simulink model "fake_config"  (R2017b)
settings: Solver=VariableStepAuto  StartTime=0.0  StopTime=10.0  RelTol=1e-3
libraries: simulink_extras x18
(part 1 of 4)
settings Model: Creator=Tonno  LastModifiedBy=Tonno

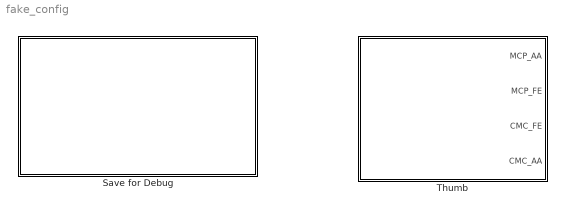
== system fake_config ==
  Save for Debug : Subsystem
  Thumb : Subsystem

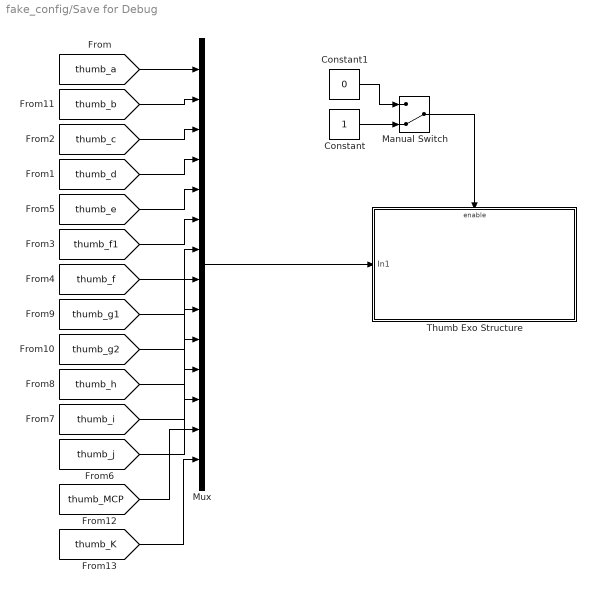
== system fake_config/Save for Debug ==
  Constant : Constant
  Constant1 : Constant  Value=0
  Manual Switch : ManualSwitch  CurrentSetting=0
  Mux : Mux  Inputs=14
  Thumb Exo Structure : Subsystem
  wires:
  Manual Switch/1 -> Thumb Exo Structure/Enable
  Constant/1 -> Manual Switch/2
  Constant1/1 -> Manual Switch/1
  [thumb_i] -> Mux/11
  [thumb_g2] -> Mux/9
  [thumb_c] -> Mux/3
  [thumb_d] -> Mux/4
  [thumb_f] -> Mux/7
  [thumb_f1] -> Mux/6
  [thumb_h] -> Mux/10
  [thumb_b] -> Mux/2
  Mux/1 -> Thumb Exo Structure/1(In1)
  [thumb_j] -> Mux/12
  [thumb_a] -> Mux/1
  [thumb_e] -> Mux/5
  [thumb_g1] -> Mux/8
  [thumb_MCP] -> Mux/13
  [thumb_K] -> Mux/14

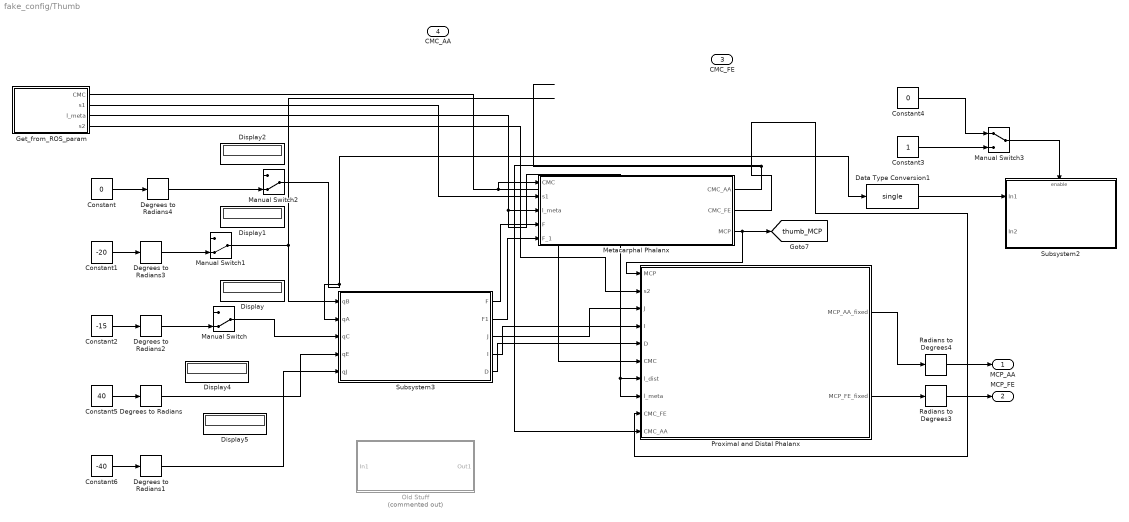
== system fake_config/Thumb ==
  Constant : Constant  Value=0
  Constant1 : Constant  Value=-20
  Constant2 : Constant  Value=-15
  Constant3 : Constant
  Constant4 : Constant  Value=0
  Constant5 : Constant  Value=40
  Constant6 : Constant  Value=-40
  Data Type Conversion1 : DataTypeConversion  OutDataTypeStr=single
  Degrees to Radians{,1..4} (5 alike) : simulink_extras/Transformations/Degrees to Radians
  Display{,1..2,4..5} (5 alike) : Display
  Get_from_ROS_param : Subsystem
  Manual Switch : ManualSwitch  CurrentSetting=0
  Manual Switch1 : ManualSwitch  CurrentSetting=0
  Manual Switch2 : ManualSwitch  CurrentSetting=0
  Manual Switch3 : ManualSwitch
  Metacarphal Phalanx : Subsystem
  Old Stuff : Subsystem  Commented=on
  Proximal and Distal Phalanx : Subsystem
  Radians to Degrees3 : simulink_extras/Transformations/Radians to Degrees
  Radians to Degrees4 : simulink_extras/Transformations/Radians to Degrees
  Subsystem2 : Subsystem
  Subsystem3 : Subsystem
  MCP_AA : Outport
  MCP_FE : Outport  Port=2
  CMC_FE : Outport  Port=3
  CMC_AA : Outport  Port=4
  tag scope: thumb_MCP=global
  wires:
  Constant2/1 -> Degrees to Radians2/1
  Constant1/1 -> Degrees to Radians3/1
  Constant/1 -> Degrees to Radians4/1
  Get_from_ROS_param/1(CMC) -> Proximal and Distal Phalanx/6(CMC), Metacarphal Phalanx/1(CMC)
  Get_from_ROS_param/2(s1) -> Metacarphal Phalanx/2(s1)
  Metacarphal Phalanx/3(MCP) -> [thumb_MCP], Proximal and Distal Phalanx/1("MCP ")
  Get_from_ROS_param/3(l_meta) -> Proximal and Distal Phalanx/7(l_dist), Proximal and Distal Phalanx/8(l_meta), Metacarphal Phalanx/3(l_meta)
  Get_from_ROS_param/4(s2) -> Proximal and Distal Phalanx/2(s2)
  Proximal and Distal Phalanx/1(MCP_AA_fixed) -> Radians to Degrees4/1
  Radians to Degrees3/1 -> MCP_FE/1
  Proximal and Distal Phalanx/2(MCP_FE_fixed) -> Radians to Degrees3/1
  Radians to Degrees4/1 -> MCP_AA/1
  Manual Switch2/1 -> Data Type Conversion1/1, Subsystem3/2(qA)
  Manual Switch1/1 -> Subsystem3/1(qB)
  Metacarphal Phalanx/2(CMC_FE) -> Proximal and Distal Phalanx/9(CMC_FE)
  Metacarphal Phalanx/1("CMC_AA ") -> Proximal and Distal Phalanx/10(CMC_AA)
  Manual Switch3/1 -> Subsystem2/Enable
  Constant3/1 -> Manual Switch3/2
  Constant4/1 -> Manual Switch3/1
  Data Type Conversion1/1 -> Subsystem2/1(In1)
  Manual Switch/1 -> Subsystem3/3(qC)
  Subsystem3/1(F) -> Metacarphal Phalanx/4(F)
  Subsystem3/2(F1) -> Metacarphal Phalanx/5(F_1)
  Subsystem3/3(J) -> Proximal and Distal Phalanx/3(J)
  Subsystem3/4(I) -> Proximal and Distal Phalanx/4(I)
  Subsystem3/5(D) -> Proximal and Distal Phalanx/5(D)
  ? -> CMC_FE/1
  ? -> CMC_AA/1
  Constant5/1 -> Degrees to Radians/1
  Constant6/1 -> Degrees to Radians1/1
  Degrees to Radians1/1 -> Subsystem3/5(qJ)
  Degrees to Radians/1 -> Subsystem3/4(qE)
  Degrees to Radians2/1 -> Manual Switch/2
  Degrees to Radians3/1 -> Manual Switch1/2
  Degrees to Radians4/1 -> Manual Switch2/2

== system fake_config/Save for Debug/Thumb Exo Structure ==
  In1 : Inport
  Enable : EnablePort
  Data Type Conversion1 : DataTypeConversion  OutDataTypeStr=double
  To File : ToFile  Filename=exo_points.mat  MatrixName=points
  wires:
  In1/1 -> Data Type Conversion1/1
  Data Type Conversion1/1 -> To File/1

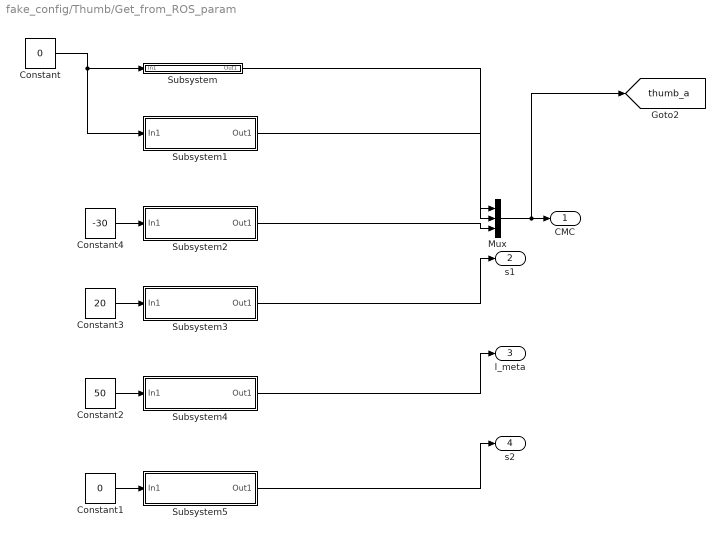
== system fake_config/Thumb/Get_from_ROS_param ==
  Constant : Constant  Value=0
  Constant1 : Constant  Value=0
  Constant2 : Constant  Value=50
  Constant3 : Constant  Value=20
  Constant4 : Constant  Value=-30
  Mux : Mux  Inputs=3
  Subsystem : Subsystem
  Subsystem1 : Subsystem
  Subsystem2 : Subsystem
  Subsystem3 : Subsystem
  Subsystem4 : Subsystem
  Subsystem5 : Subsystem
  CMC : Outport
  s1 : Outport  Port=2
  l_meta : Outport  Port=3
  s2 : Outport  Port=4
  tag scope: thumb_a=global
  wires:
  Mux/1 -> [thumb_a], CMC/1
  Subsystem/1(Out1) -> Mux/1
  Subsystem1/1(Out1) -> Mux/2
  Subsystem2/1(Out1) -> Mux/3
  Subsystem3/1(Out1) -> s1/1
  Subsystem4/1(Out1) -> l_meta/1
  Subsystem5/1(Out1) -> s2/1
  Constant/1 -> Subsystem1/1(In1), Subsystem/1(In1)
  Constant3/1 -> Subsystem3/1(In1)
  Constant2/1 -> Subsystem4/1(In1)
  Constant1/1 -> Subsystem5/1(In1)
  Constant4/1 -> Subsystem2/1(In1)

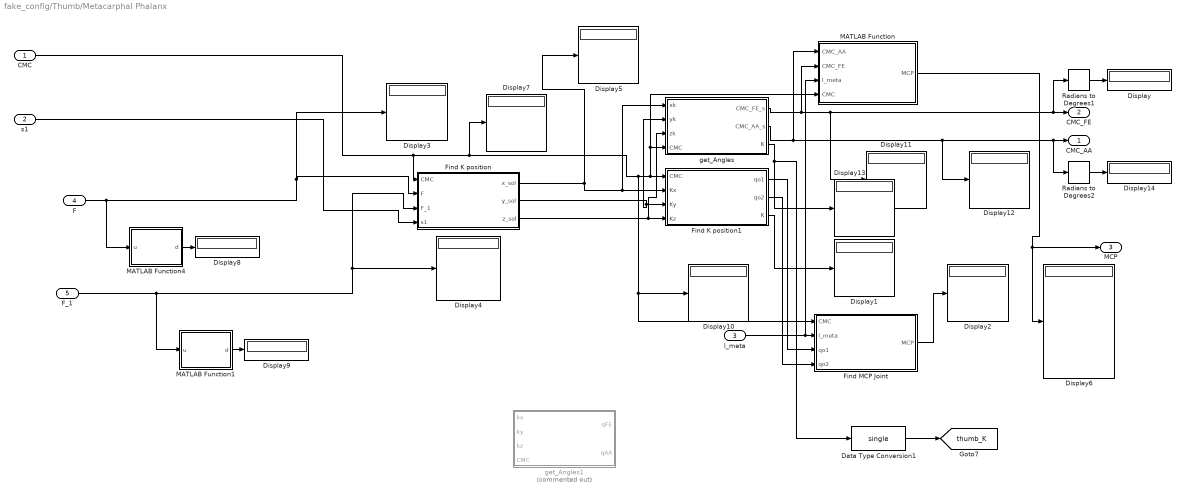
== system fake_config/Thumb/Metacarphal Phalanx ==
  CMC : Inport
  s1 : Inport  Port=2
  l_meta : Inport  Port=3
  F : Inport  Port=4
  F_1 : Inport  Port=5
  Data Type Conversion1 : DataTypeConversion  OutDataTypeStr=single
  Display{,1..14} (15 alike) : Display
  Find K position : MATLAB Function  TreatAsAtomicUnit=on
  Find K position1 : MATLAB Function  TreatAsAtomicUnit=on
  Find MCP Joint : MATLAB Function  TreatAsAtomicUnit=on
  MATLAB Function : MATLAB Function  TreatAsAtomicUnit=on
  MATLAB Function1 : MATLAB Function  TreatAsAtomicUnit=on
  MATLAB Function4 : MATLAB Function  TreatAsAtomicUnit=on
  Radians to Degrees1 : simulink_extras/Transformations/Radians to Degrees
  Radians to Degrees2 : simulink_extras/Transformations/Radians to Degrees
  get_Angles : MATLAB Function  TreatAsAtomicUnit=on
  get_Angles1 : MATLAB Function  Commented=on  TreatAsAtomicUnit=on
  "CMC_AA " : Outport
  CMC_FE : Outport  Port=2
  MCP : Outport  Port=3
  tag scope: thumb_K=global
  wires:
  Find K position/2(y_sol) -> get_Angles/2(yk), Find K position1/3(Ky)
  Find K position1/1(qo1) -> Find MCP Joint/3(qo1)
  Find K position1/2(qo2) -> Find MCP Joint/4(qo2)
  Find K position/3(z_sol) -> get_Angles/3(zk), Find K position1/4(Kz)
  Find K position/1(x_sol) -> Display5/1, get_Angles/1(xk), Find K position1/2(Kx)
  CMC/1 -> Display7/1, Display10/1, Find MCP Joint/1(CMC), MATLAB Function/4(CMC), get_Angles/4(CMC), Find K position1/1(CMC), Find K position/1(CMC)
  s1/1 -> Find K position/4(s1)
  l_meta/1 -> MATLAB Function/3(l_meta), Find MCP Joint/2(l_meta)
  Find MCP Joint/1(MCP) -> Display2/1
  Find K position1/3(K) -> Display1/1
  get_Angles/2(CMC_AA_s) -> MATLAB Function/1(CMC_AA), Display12/1, Radians to Degrees2/1, "CMC_AA "/1
  get_Angles/1(CMC_FE_s) -> MATLAB Function/2(CMC_FE), Display11/1, Radians to Degrees1/1, CMC_FE/1
  MATLAB Function4/1(d) -> Display8/1
  F/1 -> MATLAB Function4/1(u), Find K position/2(F), Display3/1
  MATLAB Function1/1(d) -> Display9/1
  F_1/1 -> MATLAB Function1/1(u), Find K position/3(F_1), Display4/1
  MATLAB Function/1(MCP) -> MCP/1, Display6/1
  get_Angles/3(K) -> Data Type Conversion1/1, Display13/1
  Radians to Degrees1/1 -> Display/1
  Radians to Degrees2/1 -> Display14/1
  Data Type Conversion1/1 -> [thumb_K]

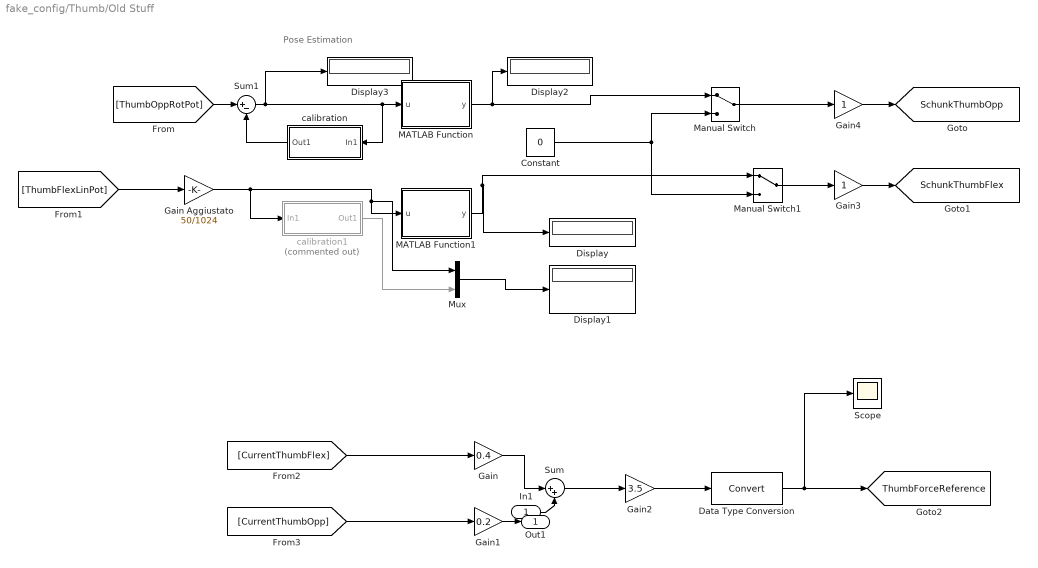
== system fake_config/Thumb/Old Stuff ==
  note: Pose Estimation
  In1 : Inport
  Constant : Constant  Value=0  OutDataTypeStr=single
  Data Type Conversion : DataTypeConversion
  Display{,1..3} (4 alike) : Display
  Gain : Gain  Gain=0.4
  Gain Aggiustato : Gain  Gain=50/1024
  Gain1 : Gain  Gain=0.2
  Gain2 : Gain  Gain=3.5
  Gain3 : Gain
  Gain4 : Gain
  MATLAB Function : MATLAB Function  TreatAsAtomicUnit=on
  MATLAB Function1 : MATLAB Function  TreatAsAtomicUnit=on
  Manual Switch : ManualSwitch
  Manual Switch1 : ManualSwitch
  Mux : Mux  Inputs=2
  Scope : Scope
  Sum : Sum  Inputs=|++
  Sum1 : Sum  Inputs=|+-
  calibration : Subsystem
  calibration1 : Subsystem  Commented=on
  Out1 : Outport
  tag scope: SchunkThumbFlex=global, SchunkThumbOpp=global, ThumbForceReference=global
  wires:
  Gain1/1 -> Out1/1
  In1/1 -> Sum/2
  MATLAB Function/1(y) -> Display2/1, Manual Switch/1
  Gain4/1 -> [SchunkThumbOpp]
  [ThumbFlexLinPot] -> Gain Aggiustato/1
  Sum/1 -> Gain2/1
  Data Type Conversion/1 -> Scope/1, [ThumbForceReference]
  Gain2/1 -> Data Type Conversion/1
  Gain3/1 -> [SchunkThumbFlex]
  Sum1/1 -> Display3/1, calibration/1(In1), MATLAB Function/1(u)
  Mux/1 -> Display1/1
  [CurrentThumbFlex] -> Gain/1
  MATLAB Function1/1(y) -> Manual Switch1/1, Display/1
  Manual Switch/1 -> Gain4/1
  Manual Switch1/1 -> Gain3/1
  [CurrentThumbOpp] -> Gain1/1
  Constant/1 -> Manual Switch1/2, Manual Switch/2
  calibration/1(Out1) -> Sum1/2
  Gain/1 -> Sum/1
  calibration1/1(Out1) -> Mux/2
  Gain Aggiustato/1 -> calibration1/1(In1), Mux/1, MATLAB Function1/1(u)
  [ThumbOppRotPot] -> Sum1/1

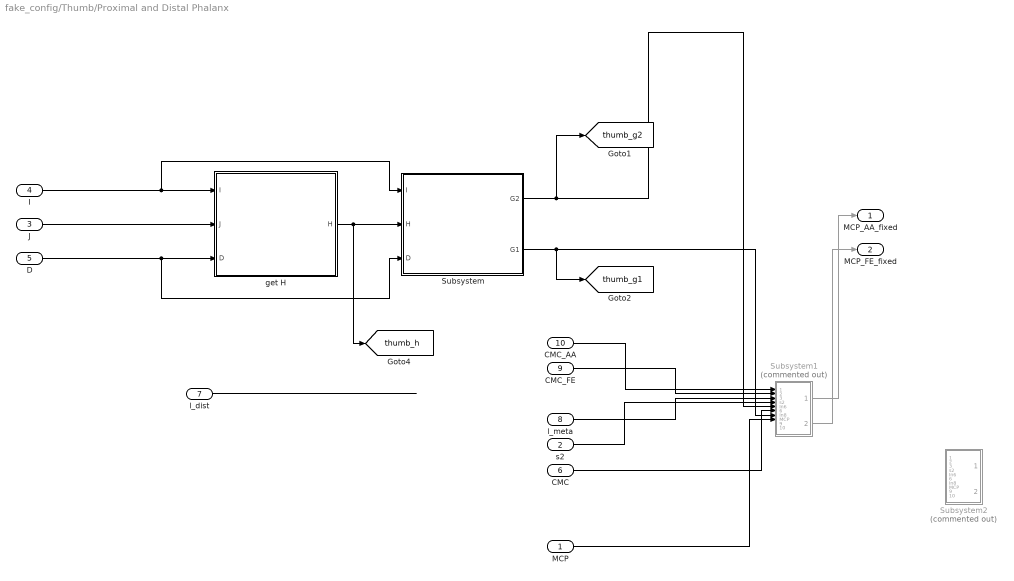
== system fake_config/Thumb/Proximal and Distal Phalanx ==
  "MCP " : Inport
  s2 : Inport  Port=2
  J : Inport  Port=3
  I : Inport  Port=4
  D : Inport  Port=5
  CMC : Inport  Port=6
  l_dist : Inport  Port=7
  l_meta : Inport  Port=8
  CMC_FE : Inport  Port=9
  CMC_AA : Inport  Port=10
  Subsystem : Subsystem
  Subsystem1 : Subsystem  Commented=on
  Subsystem2 : Subsystem  Commented=on
  get H : Subsystem
  MCP_AA_fixed : Outport
  MCP_FE_fixed : Outport  Port=2
  tag scope: thumb_g1=global, thumb_g2=global, thumb_h=global
  wires:
  I/1 -> Subsystem/1(I), get H/1(I)
  J/1 -> get H/2(J)
  D/1 -> Subsystem/3(D), get H/3(D)
  get H/1(H) -> [thumb_h], Subsystem/2(H)
  CMC_AA/1 -> Subsystem1/1(CMC_AA)
  CMC_FE/1 -> Subsystem1/2(CMC_FE)
  l_dist/1 -> ?
  l_meta/1 -> Subsystem1/3(l_meta)
  s2/1 -> Subsystem1/4(s2)
  Subsystem/1(G2) -> [thumb_g2], Subsystem1/5(In6)
  CMC/1 -> Subsystem1/6(CMC)
  Subsystem/2(G1) -> [thumb_g1], Subsystem1/7(In8)
  "MCP "/1 -> Subsystem1/8("MCP ")
  Subsystem1/1(MCP_AA_fixed) -> MCP_AA_fixed/1
  Subsystem1/2(MCP_FE_fixed) -> MCP_FE_fixed/1

== system fake_config/Thumb/Subsystem2 ==
  In1 : Inport
  In2 : Inport  Port=2
  Enable : EnablePort
  Data Type Conversion1 : DataTypeConversion  OutDataTypeStr=double
  Mux : Mux  Inputs=2
  To File : ToFile  Filename=thumb_force.mat  MatrixName=forza_gravita
  wires:
  In1/1 -> Mux/1
  Mux/1 -> Data Type Conversion1/1
  In2/1 -> Mux/2
  Data Type Conversion1/1 -> To File/1

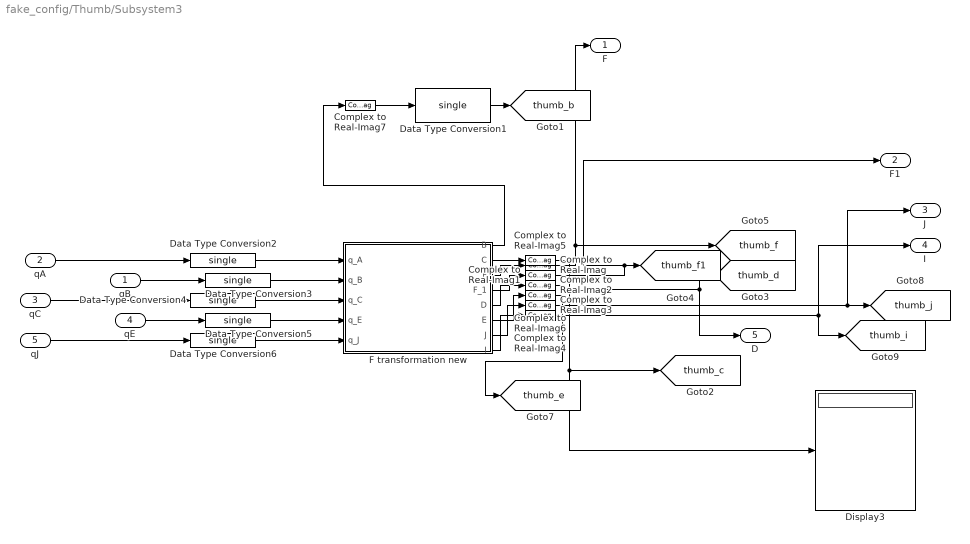
== system fake_config/Thumb/Subsystem3 ==
  qB : Inport
  qA : Inport  Port=2
  qC : Inport  Port=3
  qE : Inport  Port=4
  qJ : Inport  Port=5
  Complex to Real-Imag{,1..7} (8 alike) : ComplexToRealImag  Output=Real
  Data Type Conversion{1..6} (6 alike) : DataTypeConversion  OutDataTypeStr=single
  Display3 : Display
  F transformation new : MATLAB Function  TreatAsAtomicUnit=on
  F : Outport
  F1 : Outport  Port=2
  J : Outport  Port=3
  I : Outport  Port=4
  D : Outport  Port=5
  tag scope: thumb_b=global, thumb_c=global, thumb_d=global, thumb_e=global, thumb_f1=global, thumb_f=global, thumb_i=global, thumb_j=global
  wires:
  Complex to Real-Imag5/1 -> Display3/1, [thumb_c]
  qA/1 -> Data Type Conversion2/1
  Complex to Real-Imag6/1 -> [thumb_e]
  F transformation new/6(E) -> Complex to Real-Imag6/1
  F transformation new/1(B) -> Complex to Real-Imag7/1
  qE/1 -> Data Type Conversion5/1
  qB/1 -> Data Type Conversion3/1
  qC/1 -> Data Type Conversion4/1
  F transformation new/3(F) -> Complex to Real-Imag/1
  F transformation new/4(F_1) -> Complex to Real-Imag1/1
  F transformation new/7(J) -> Complex to Real-Imag3/1
  F transformation new/8(I) -> Complex to Real-Imag4/1
  F transformation new/5(D) -> Complex to Real-Imag2/1
  Complex to Real-Imag/1 -> F/1, [thumb_f]
  Complex to Real-Imag1/1 -> F1/1, [thumb_f1]
  Complex to Real-Imag2/1 -> D/1, [thumb_d]
  Complex to Real-Imag3/1 -> J/1, [thumb_j]
  Complex to Real-Imag4/1 -> I/1, [thumb_i]
  F transformation new/2(C) -> Complex to Real-Imag5/1
  Complex to Real-Imag7/1 -> Data Type Conversion1/1
  Data Type Conversion1/1 -> [thumb_b]
  Data Type Conversion2/1 -> F transformation new/1(q_A)
  Data Type Conversion3/1 -> F transformation new/2(q_B)
  Data Type Conversion4/1 -> F transformation new/3(q_C)
  Data Type Conversion5/1 -> F transformation new/4(q_E)
  Data Type Conversion6/1 -> F transformation new/5(q_J)
  qJ/1 -> Data Type Conversion6/1

== system fake_config/Thumb/Get_from_ROS_param/Subsystem ==
  In1 : Inport
  Data Type Conversion1 : DataTypeConversion  OutDataTypeStr=single
  Rate Transition : RateTransition  InitialCondition=-10.0
  Out1 : Outport
  wires:
  Data Type Conversion1/1 -> Out1/1
  In1/1 -> Rate Transition/1
  Rate Transition/1 -> Data Type Conversion1/1

== system fake_config/Thumb/Get_from_ROS_param/Subsystem1 ==
  In1 : Inport
  Data Type Conversion1 : DataTypeConversion  OutDataTypeStr=single
  Rate Transition : RateTransition  InitialCondition=0.0
  Out1 : Outport
  wires:
  Data Type Conversion1/1 -> Out1/1
  In1/1 -> Rate Transition/1
  Rate Transition/1 -> Data Type Conversion1/1

== system fake_config/Thumb/Get_from_ROS_param/Subsystem2 ==
  In1 : Inport
  Data Type Conversion1 : DataTypeConversion  OutDataTypeStr=single
  Rate Transition : RateTransition  InitialCondition=-32.0
  Out1 : Outport
  wires:
  Data Type Conversion1/1 -> Out1/1
  In1/1 -> Rate Transition/1
  Rate Transition/1 -> Data Type Conversion1/1

== system fake_config/Thumb/Get_from_ROS_param/Subsystem3 ==
  In1 : Inport
  Data Type Conversion1 : DataTypeConversion  OutDataTypeStr=single
  Rate Transition : RateTransition  InitialCondition=20.0
  Out1 : Outport
  wires:
  Data Type Conversion1/1 -> Out1/1
  In1/1 -> Rate Transition/1
  Rate Transition/1 -> Data Type Conversion1/1

== system fake_config/Thumb/Get_from_ROS_param/Subsystem4 ==
  In1 : Inport
  Data Type Conversion1 : DataTypeConversion  OutDataTypeStr=single
  Rate Transition : RateTransition  InitialCondition=50.0
  Out1 : Outport
  wires:
  Data Type Conversion1/1 -> Out1/1
  In1/1 -> Rate Transition/1
  Rate Transition/1 -> Data Type Conversion1/1

== system fake_config/Thumb/Get_from_ROS_param/Subsystem5 ==
  In1 : Inport
  Data Type Conversion1 : DataTypeConversion  OutDataTypeStr=single
  Rate Transition : RateTransition  InitialCondition=20.0
  Out1 : Outport
  wires:
  Data Type Conversion1/1 -> Out1/1
  In1/1 -> Rate Transition/1
  Rate Transition/1 -> Data Type Conversion1/1

== system fake_config/Thumb/Old Stuff/calibration ==
  In1 : Inport
  Constant2 : Constant  Value=540  OutDataTypeStr=single
  Constant3 : Constant  Value=540  OutDataTypeStr=single
  Display4 : Display
  Subsystem : Subsystem
  Sum2 : Sum  Inputs=|++
  Switch : Switch  Criteria=u2 > Threshold
  Out1 : Outport
  wires:
  [CalibrationSignal] -> Switch/2
  Subsystem/1(Out1) -> Switch/3
  Constant3/1 -> Sum2/1
  [CalibrationSignal] -> Subsystem/Enable
  Constant2/1 -> Switch/1
  Sum2/1 -> Display4/1, Subsystem/1(In1)
  In1/1 -> Sum2/2
  Switch/1 -> Out1/1

== system fake_config/Thumb/Old Stuff/calibration1 ==
  In1 : Inport
  Subsystem1 : Subsystem
  Out1 : Outport
  wires:
  [CalibrationSignal] -> Subsystem1/Enable
  In1/1 -> Subsystem1/1(In1)
  Subsystem1/1(Out1) -> Out1/1

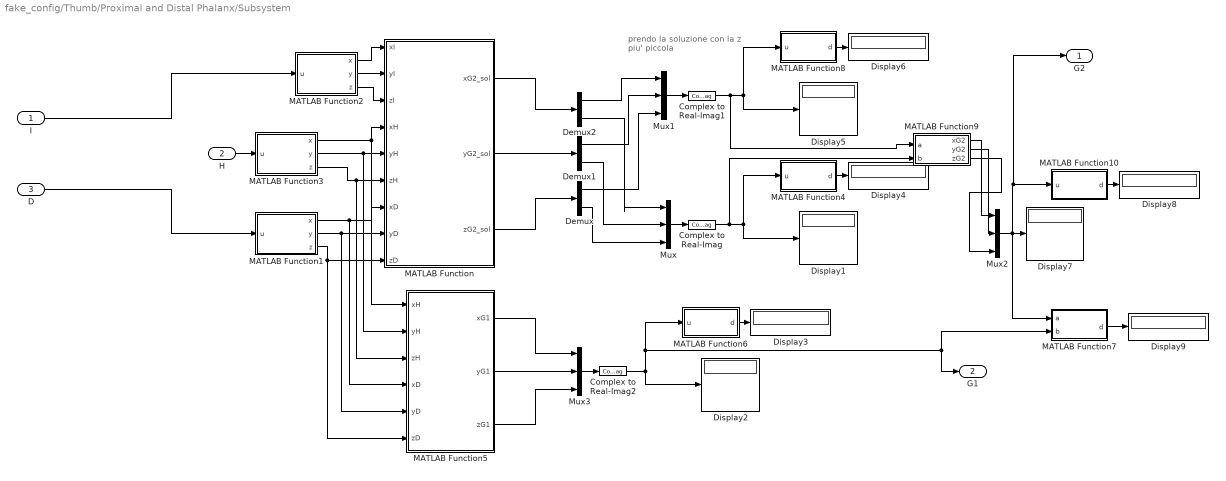
== system fake_config/Thumb/Proximal and Distal Phalanx/Subsystem ==
  note: prendo la soluzione
      | con la z piu' piccola
  I : Inport
  H : Inport  Port=2
  D : Inport  Port=3
  Complex to Real-Imag : ComplexToRealImag  Output=Real
  Complex to Real-Imag1 : ComplexToRealImag  Output=Real
  Complex to Real-Imag2 : ComplexToRealImag  Output=Real
  Demux : Demux  Outputs=2
  Demux1 : Demux  Outputs=2
  Demux2 : Demux  Outputs=2
  Display{1..9} (9 alike) : Display
  MATLAB Function : MATLAB Function  TreatAsAtomicUnit=on
  MATLAB Function1 : MATLAB Function  TreatAsAtomicUnit=on
  MATLAB Function10 : MATLAB Function  TreatAsAtomicUnit=on
  MATLAB Function2 : MATLAB Function  TreatAsAtomicUnit=on
  MATLAB Function3 : MATLAB Function  TreatAsAtomicUnit=on
  MATLAB Function4 : MATLAB Function  TreatAsAtomicUnit=on
  MATLAB Function5 : MATLAB Function  TreatAsAtomicUnit=on
  MATLAB Function6 : MATLAB Function  TreatAsAtomicUnit=on
  MATLAB Function7 : MATLAB Function  TreatAsAtomicUnit=on
  MATLAB Function8 : MATLAB Function  TreatAsAtomicUnit=on
  MATLAB Function9 : MATLAB Function  TreatAsAtomicUnit=on
  Mux{,1..3} (4 alike) : Mux  Inputs=3
  G2 : Outport
  G1 : Outport  Port=2
  wires:
  MATLAB Function1/2(y) -> MATLAB Function/8(yD), MATLAB Function5/5(yD)
  H/1 -> MATLAB Function3/1(u)
  MATLAB Function3/1(x) -> MATLAB Function5/1(xH), MATLAB Function/4(xH)
  MATLAB Function2/1(x) -> MATLAB Function/1(xI)
  D/1 -> MATLAB Function1/1(u)
  MATLAB Function/1(xG2_sol) -> Demux2/1
  Complex to Real-Imag1/1 -> MATLAB Function9/1(a), Display5/1, MATLAB Function8/1(u)
  Demux/2 -> Mux/3
  MATLAB Function10/1(d) -> Display8/1
  MATLAB Function/3(zG2_sol) -> Demux/1
  MATLAB Function2/3(z) -> MATLAB Function/3(zI)
  MATLAB Function2/2(y) -> MATLAB Function/2(yI)
  MATLAB Function9/3(zG2) -> Mux2/3
  Demux2/1 -> Mux1/1
  MATLAB Function1/3(z) -> MATLAB Function5/6(zD), MATLAB Function/9(zD)
  MATLAB Function9/1(xG2) -> Mux2/1
  Demux1/1 -> Mux1/2
  MATLAB Function1/1(x) -> MATLAB Function/7(xD), MATLAB Function5/4(xD)
  Complex to Real-Imag/1 -> MATLAB Function9/2(b), Display1/1, MATLAB Function4/1(u)
  Demux2/2 -> Mux/1
  MATLAB Function9/2(yG2) -> Mux2/2
  I/1 -> MATLAB Function2/1(u)
  Demux/1 -> Mux1/3
  Mux1/1 -> Complex to Real-Imag1/1
  Mux/1 -> Complex to Real-Imag/1
  MATLAB Function3/2(y) -> MATLAB Function5/2(yH), MATLAB Function/5(yH)
  MATLAB Function4/1(d) -> Display4/1
  MATLAB Function3/3(z) -> MATLAB Function/6(zH), MATLAB Function5/3(zH)
  Demux1/2 -> Mux/2
  MATLAB Function/2(yG2_sol) -> Demux1/1
  MATLAB Function8/1(d) -> Display6/1
  Mux3/1 -> Complex to Real-Imag2/1
  MATLAB Function5/2(yG1) -> Mux3/2
  MATLAB Function5/1(xG1) -> Mux3/1
  MATLAB Function5/3(zG1) -> Mux3/3
  MATLAB Function6/1(d) -> Display3/1
  Complex to Real-Imag2/1 -> Display2/1, G1/1, MATLAB Function7/2(b), MATLAB Function6/1(u)
  Mux2/1 -> MATLAB Function7/1(a), G2/1, MATLAB Function10/1(u), Display7/1
  MATLAB Function7/1(d) -> Display9/1

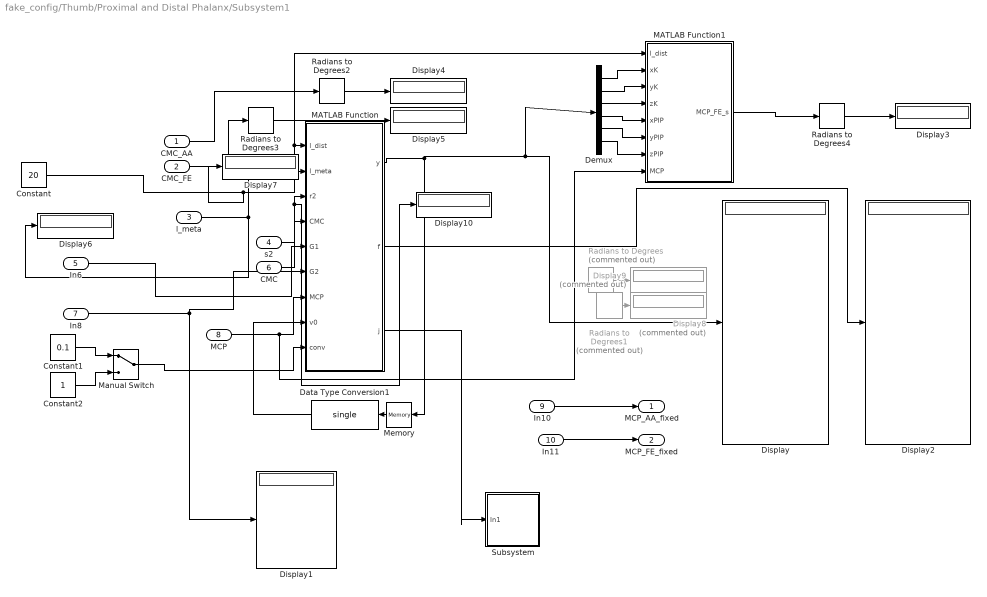
== system fake_config/Thumb/Proximal and Distal Phalanx/Subsystem1 ==
  CMC_AA : Inport
  CMC_FE : Inport  Port=2
  l_meta : Inport  Port=3
  s2 : Inport  Port=4
  In6 : Inport  Port=5
  CMC : Inport  Port=6
  In8 : Inport  Port=7
  "MCP " : Inport  Port=8
  In10 : Inport  Port=9
  In11 : Inport  Port=10
  Constant : Constant  Value=20  OutDataTypeStr=single
  Constant1 : Constant  Value=0.1  OutDataTypeStr=single
  Constant2 : Constant  OutDataTypeStr=single
  Data Type Conversion1 : DataTypeConversion  OutDataTypeStr=single
  Demux : Demux  Outputs=6
  Display{,1..7,10} (9 alike) : Display
  Display8 : Display  Commented=on
  Display9 : Display  Commented=on
  MATLAB Function : MATLAB Function  TreatAsAtomicUnit=on
  MATLAB Function1 : MATLAB Function  TreatAsAtomicUnit=on
  Manual Switch : ManualSwitch
  Memory : Memory
  Radians to Degrees : simulink_extras/Transformations/Radians to Degrees  Commented=on
  Radians to Degrees1 : simulink_extras/Transformations/Radians to Degrees  Commented=on
  Radians to Degrees2 : simulink_extras/Transformations/Radians to Degrees
  Radians to Degrees3 : simulink_extras/Transformations/Radians to Degrees
  Radians to Degrees4 : simulink_extras/Transformations/Radians to Degrees
  Subsystem : Subsystem
  MCP_AA_fixed : Outport
  MCP_FE_fixed : Outport  Port=2
  wires:
  ? -> Radians to Degrees1/1
  MATLAB Function/2(f) -> Display2/1
  Memory/1 -> Data Type Conversion1/1
  Data Type Conversion1/1 -> MATLAB Function/8(v0)
  Radians to Degrees1/1 -> Display8/1
  CMC_AA/1 -> Radians to Degrees2/1
  MATLAB Function/1(y) -> Demux/1, Display/1, Memory/1
  Radians to Degrees/1 -> Display9/1
  s2/1 -> Display10/1, MATLAB Function/3(r2)
  In8/1 -> MATLAB Function/6(G2), Display1/1
  CMC_FE/1 -> Radians to Degrees3/1
  "MCP "/1 -> MATLAB Function1/8(MCP), MATLAB Function/7(MCP)
  ? -> Radians to Degrees/1
  In10/1 -> MCP_AA_fixed/1
  In11/1 -> MCP_FE_fixed/1
  In6/1 -> MATLAB Function/5(G1)
  CMC/1 -> MATLAB Function/4(CMC)
  l_meta/1 -> Display6/1, MATLAB Function/2(l_meta)
  Constant/1 -> Display7/1, MATLAB Function1/1(l_dist), MATLAB Function/1(l_dist)
  MATLAB Function/3(j) -> Subsystem/1(In1)
  Radians to Degrees2/1 -> Display4/1
  Radians to Degrees3/1 -> Display5/1
  MATLAB Function1/1(MCP_FE_s) -> Radians to Degrees4/1
  Demux/6 -> MATLAB Function1/7(zPIP)
  Demux/5 -> MATLAB Function1/6(yPIP)
  Demux/4 -> MATLAB Function1/5(xPIP)
  Demux/3 -> MATLAB Function1/4(zK)
  Demux/2 -> MATLAB Function1/3(yK)
  Demux/1 -> MATLAB Function1/2(xK)
  Radians to Degrees4/1 -> Display3/1
  Manual Switch/1 -> MATLAB Function/9(conv)
  Constant1/1 -> Manual Switch/1
  Constant2/1 -> Manual Switch/2

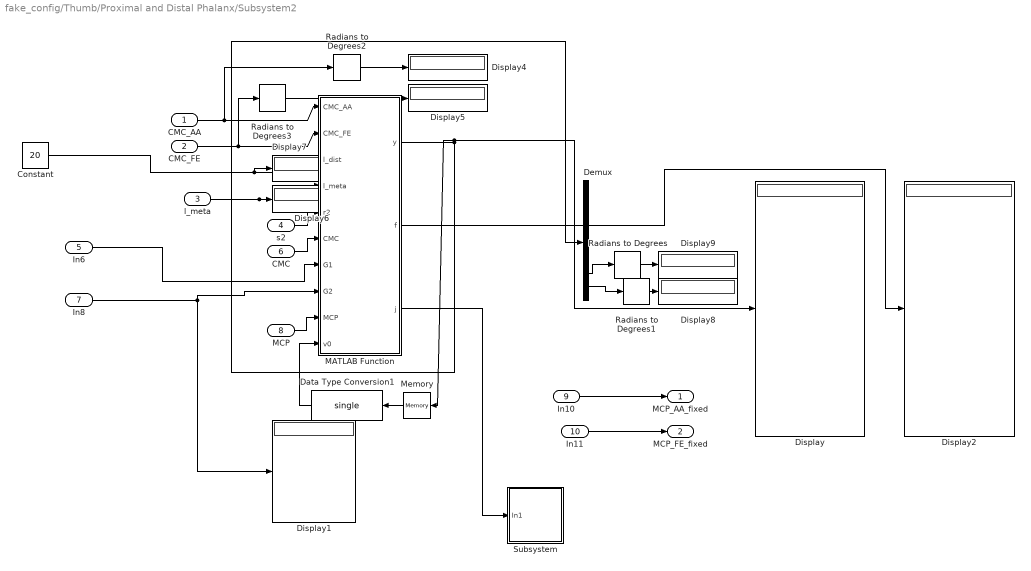
== system fake_config/Thumb/Proximal and Distal Phalanx/Subsystem2 ==
  CMC_AA : Inport
  CMC_FE : Inport  Port=2
  l_meta : Inport  Port=3
  s2 : Inport  Port=4
  In6 : Inport  Port=5
  CMC : Inport  Port=6
  In8 : Inport  Port=7
  "MCP " : Inport  Port=8
  In10 : Inport  Port=9
  In11 : Inport  Port=10
  Constant : Constant  Value=20  OutDataTypeStr=single
  Data Type Conversion1 : DataTypeConversion  OutDataTypeStr=single
  Demux : Demux  Outputs=8
  Display{,1..2,4..9} (9 alike) : Display
  MATLAB Function : MATLAB Function  TreatAsAtomicUnit=on
  Memory : Memory
  Radians to Degrees{,1..3} (4 alike) : simulink_extras/Transformations/Radians to Degrees
  Subsystem : Subsystem
  MCP_AA_fixed : Outport
  MCP_FE_fixed : Outport  Port=2
  wires:
  Demux/8 -> Radians to Degrees1/1
  MATLAB Function/2(f) -> Display2/1
  Memory/1 -> Data Type Conversion1/1
  Data Type Conversion1/1 -> MATLAB Function/10(v0)
  Radians to Degrees1/1 -> Display8/1
  CMC_AA/1 -> Radians to Degrees2/1, MATLAB Function/1(CMC_AA)
  MATLAB Function/1(y) -> Memory/1, Display/1, Demux/1
  Radians to Degrees/1 -> Display9/1
  s2/1 -> MATLAB Function/5(r2)
  In8/1 -> MATLAB Function/8(G2), Display1/1
  CMC_FE/1 -> Radians to Degrees3/1, MATLAB Function/2(CMC_FE)
  "MCP "/1 -> MATLAB Function/9(MCP)
  Demux/7 -> Radians to Degrees/1
  In10/1 -> MCP_AA_fixed/1
  In11/1 -> MCP_FE_fixed/1
  In6/1 -> MATLAB Function/7(G1)
  CMC/1 -> MATLAB Function/6(CMC)
  l_meta/1 -> Display6/1, MATLAB Function/4(l_meta)
  Constant/1 -> Display7/1, MATLAB Function/3(l_dist)
  MATLAB Function/3(j) -> Subsystem/1(In1)
  Radians to Degrees2/1 -> Display4/1
  Radians to Degrees3/1 -> Display5/1

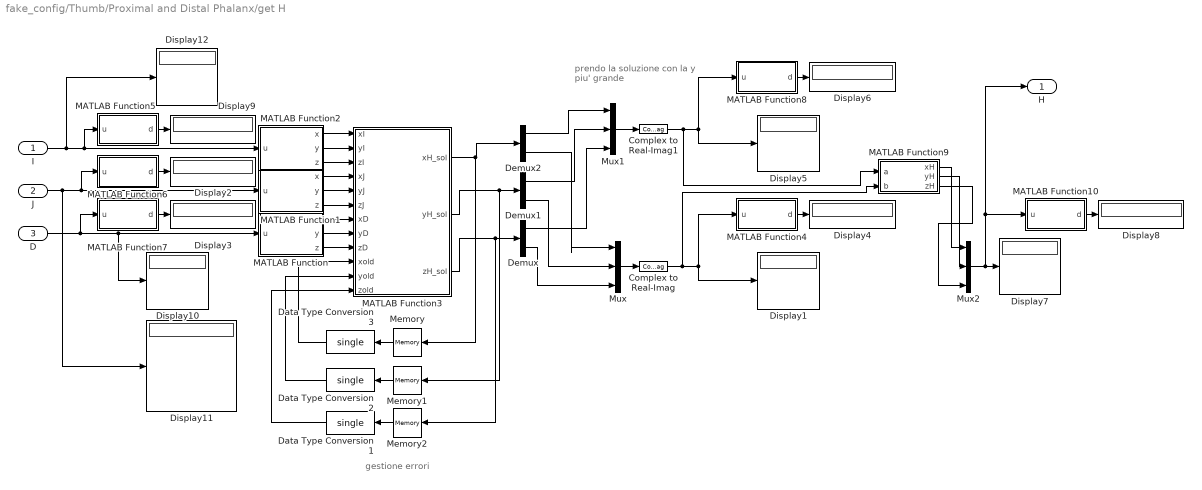
== system fake_config/Thumb/Proximal and Distal Phalanx/get H ==
  note: prendo la soluzione
      | con la y piu' grande
  note: gestione errori
  I : Inport
  J : Inport  Port=2
  D : Inport  Port=3
  Complex to Real-Imag : ComplexToRealImag  Output=Real
  Complex to Real-Imag1 : ComplexToRealImag  Output=Real
  Data Type Conversion1 : DataTypeConversion  OutDataTypeStr=single
  Data Type Conversion2 : DataTypeConversion  OutDataTypeStr=single
  Data Type Conversion3 : DataTypeConversion  OutDataTypeStr=single
  Demux : Demux  Outputs=2
  Demux1 : Demux  Outputs=2
  Demux2 : Demux  Outputs=2
  Display{1..12} (12 alike) : Display
  MATLAB Function : MATLAB Function  TreatAsAtomicUnit=on
  MATLAB Function1 : MATLAB Function  TreatAsAtomicUnit=on
  MATLAB Function10 : MATLAB Function  TreatAsAtomicUnit=on
  MATLAB Function2 : MATLAB Function  TreatAsAtomicUnit=on
  MATLAB Function3 : MATLAB Function  TreatAsAtomicUnit=on
  MATLAB Function4 : MATLAB Function  TreatAsAtomicUnit=on
  MATLAB Function5 : MATLAB Function  TreatAsAtomicUnit=on
  MATLAB Function6 : MATLAB Function  TreatAsAtomicUnit=on
  MATLAB Function7 : MATLAB Function  TreatAsAtomicUnit=on
  MATLAB Function8 : MATLAB Function  TreatAsAtomicUnit=on
  MATLAB Function9 : MATLAB Function  TreatAsAtomicUnit=on
  Memory : Memory  InitialCondition=[0,0]
  Memory1 : Memory  InitialCondition=[0,0]
  Memory2 : Memory  InitialCondition=[0,0]
  Mux : Mux  Inputs=3
  Mux1 : Mux  Inputs=3
  Mux2 : Mux  Inputs=3
  H : Outport
  wires:
  MATLAB Function3/1(xH_sol) -> Memory/1, Demux2/1
  MATLAB Function3/2(yH_sol) -> Memory1/1, Demux1/1
  MATLAB Function9/2(yH) -> Mux2/2
  MATLAB Function9/1(xH) -> Mux2/1
  MATLAB Function4/1(d) -> Display4/1
  Mux2/1 -> H/1, MATLAB Function10/1(u), Display7/1
  Demux2/2 -> Mux/1
  MATLAB Function8/1(d) -> Display6/1
  MATLAB Function6/1(d) -> Display2/1
  MATLAB Function5/1(d) -> Display9/1
  MATLAB Function9/3(zH) -> Mux2/3
  Demux/2 -> Mux/3
  Complex to Real-Imag1/1 -> MATLAB Function9/1(a), Display5/1, MATLAB Function8/1(u)
  Complex to Real-Imag/1 -> MATLAB Function9/2(b), Display1/1, MATLAB Function4/1(u)
  MATLAB Function7/1(d) -> Display3/1
  Demux1/1 -> Mux1/2
  Mux/1 -> Complex to Real-Imag/1
  MATLAB Function10/1(d) -> Display8/1
  Demux2/1 -> Mux1/1
  Demux/1 -> Mux1/3
  MATLAB Function2/2(y) -> MATLAB Function3/2(yI)
  MATLAB Function2/1(x) -> MATLAB Function3/1(xI)
  Demux1/2 -> Mux/2
  MATLAB Function/1(x) -> MATLAB Function3/7(xD)
  D/1 -> MATLAB Function7/1(u), Display10/1, MATLAB Function/1(u)
  MATLAB Function/3(z) -> MATLAB Function3/9(zD)
  MATLAB Function/2(y) -> MATLAB Function3/8(yD)
  MATLAB Function1/1(x) -> MATLAB Function3/4(xJ)
  MATLAB Function1/3(z) -> MATLAB Function3/6(zJ)
  I/1 -> Display12/1, MATLAB Function5/1(u), MATLAB Function2/1(u)
  J/1 -> Display11/1, MATLAB Function6/1(u), MATLAB Function1/1(u)
  MATLAB Function1/2(y) -> MATLAB Function3/5(yJ)
  MATLAB Function2/3(z) -> MATLAB Function3/3(zI)
  Mux1/1 -> Complex to Real-Imag1/1
  MATLAB Function3/3(zH_sol) -> Memory2/1, Demux/1
  Memory/1 -> Data Type Conversion3/1
  Memory1/1 -> Data Type Conversion2/1
  Memory2/1 -> Data Type Conversion1/1
  Data Type Conversion1/1 -> MATLAB Function3/12(zold)
  Data Type Conversion2/1 -> MATLAB Function3/11(yold)
  Data Type Conversion3/1 -> MATLAB Function3/10(xold)

== system fake_config/Thumb/Old Stuff/calibration/Subsystem ==
  In1 : Inport
  Enable : EnablePort
  Memory : Memory
  Out1 : Outport
  wires:
  Memory/1 -> Out1/1
  In1/1 -> Memory/1

== system fake_config/Thumb/Old Stuff/calibration1/Subsystem1 ==
  In1 : Inport
  Enable : EnablePort
  Memory : Memory  InitialCondition=400
  Out1 : Outport
  wires:
  Memory/1 -> Out1/1
  In1/1 -> Memory/1

== system fake_config/Thumb/Proximal and Distal Phalanx/Subsystem1/Subsystem ==
  In1 : Inport
  Display3 : Display
  wires:
  In1/1 -> Display3/1

== system fake_config/Thumb/Proximal and Distal Phalanx/Subsystem2/Subsystem ==
  In1 : Inport
  Display3 : Display
  wires:
  In1/1 -> Display3/1

== matlab function fake_config/Thumb/Old Stuff/MATLAB Function ==
  data: u input; y output
function y = fcn(u)
%#codegen

y = u / 30;

== matlab function fake_config/Thumb/Old Stuff/MATLAB Function1 ==
  data: u input; y output
function y = fcn(u)
%#codegen

y = single( u / 25);

== matlab function fake_config/Thumb/Proximal and Distal Phalanx/get H/MATLAB Function ==
  data: x output; u input; y output; z output
function [x,y,z] = split(u)

x = u(1);
y = u(2);
z = u(3);
